simulink model "zad5"  (R2023a)
settings: Solver=VariableStepAuto  StartTime=0.0  StopTime=10  RelTol=1e-3
values from neighbouring files (symbols this model uses):
  Gz = c2d(Gs,T,'zoh')    [zad1.m]
  Kpor = acker(A,B,bieguny)    [zad4.m]
  T = 0.5    [zad1.m]    (also in zad4.mat)
settings Model: Creator=pkutyl  LastModifiedBy=pkutyl

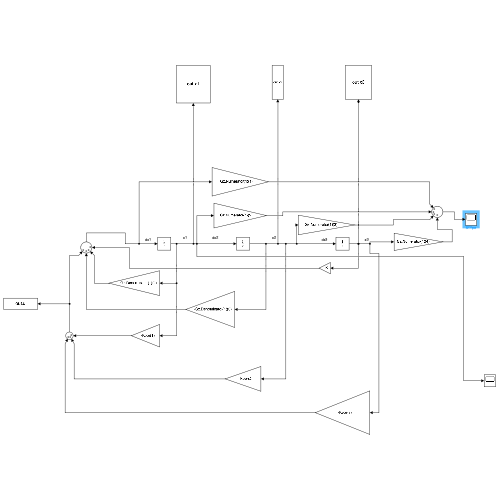
[thumbnail: Simulink's stored preview of the top-level diagram]
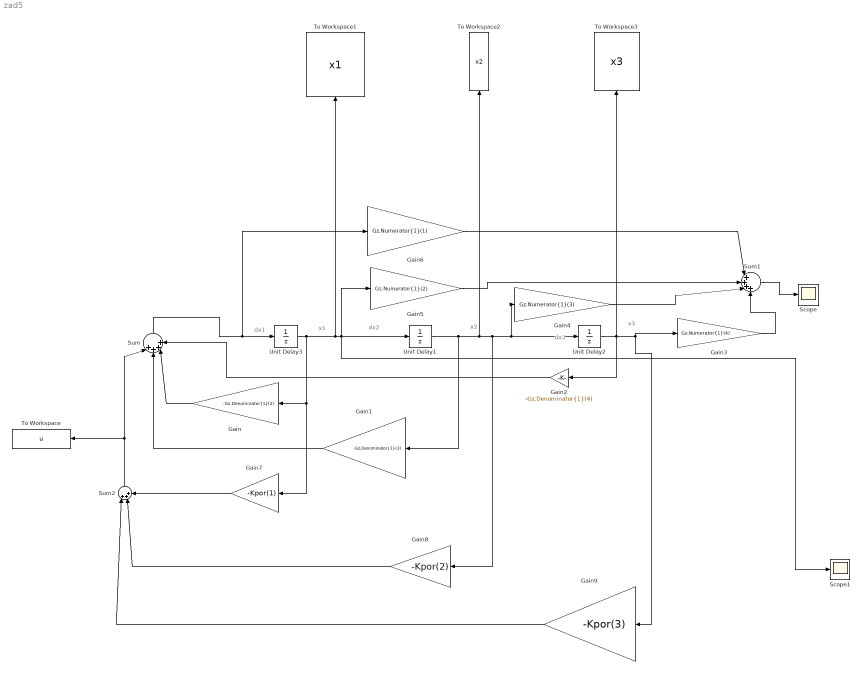
== system zad5 ==
  note: dx1
  note: dx2
  note: x1
  note: x3
  note: x2
  note: dx3
  Gain : Gain  Gain=-Gz.Denominator{1}(2)
  Gain1 : Gain  Gain=-Gz.Denominator{1}(3)
  Gain2 : Gain  Gain=-Gz.Denominator{1}(4)
  Gain3 : Gain  Gain=Gz.Numerator{1}(4)
  Gain4 : Gain  Gain=Gz.Numerator{1}(3)
  Gain5 : Gain  Gain=Gz.Numerator{1}(2)
  Gain6 : Gain  Gain=Gz.Numerator{1}(1)
  Gain7 : Gain  Gain=-Kpor(1)
  Gain8 : Gain  Gain=-Kpor(2)
  Gain9 : Gain  Gain=-Kpor(3)
  Scope : Scope
  Scope1 : Scope
  Sum : Sum  Inputs=|++++
  Sum1 : Sum  Inputs=|++++
  Sum2 : Sum  Inputs=|+++
  To Workspace : ToWorkspace  VariableName=u  SaveFormat=Structure With Time  SampleTime=-1
  To Workspace1 : ToWorkspace  VariableName=x1  SaveFormat=Structure With Time  SampleTime=-1
  To Workspace2 : ToWorkspace  VariableName=x2  SaveFormat=Structure With Time  SampleTime=-1
  To Workspace3 : ToWorkspace  VariableName=x3  SaveFormat=Structure With Time  SampleTime=-1
  Unit Delay1 : UnitDelay  InitialCondition=1  SampleTime=T  HasFrameUpgradeWarning=on
  Unit Delay2 : UnitDelay  InitialCondition=-1  SampleTime=T  HasFrameUpgradeWarning=on
  Unit Delay3 : UnitDelay  InitialCondition=2  SampleTime=T  HasFrameUpgradeWarning=on
  wires:
  Gain6/1 -> Sum1/1
  Unit Delay3/1 -> Gain7/1, Gain/1, Gain5/1, Unit Delay1/1, Scope1/1, To Workspace1/1
  Gain4/1 -> Sum1/3
  Gain9/1 -> Sum2/1
  Sum/1 -> Unit Delay3/1, Gain6/1
  Gain1/1 -> Sum/2
  Sum1/1 -> Scope/1
  Gain2/1 -> Sum/4
  Unit Delay1/1 -> Gain1/1, Gain8/1, Gain4/1, Unit Delay2/1, To Workspace2/1
  Sum2/1 -> To Workspace/1, Sum/1
  Unit Delay2/1 -> Gain3/1, Gain9/1, To Workspace3/1, Gain2/1
  Gain/1 -> Sum/3
  Gain8/1 -> Sum2/2
  Gain5/1 -> Sum1/2
  Gain7/1 -> Sum2/3
  Gain3/1 -> Sum1/4
